simulink model "VCU_CONTROL"  (R2026a)
settings: Solver=VariableStepAuto
undefined symbols (not defined in the file): VCU_torque_fall_rate, VCU_torque_rise_rate
settings Model: Creator=renil  LastModifiedBy=renil

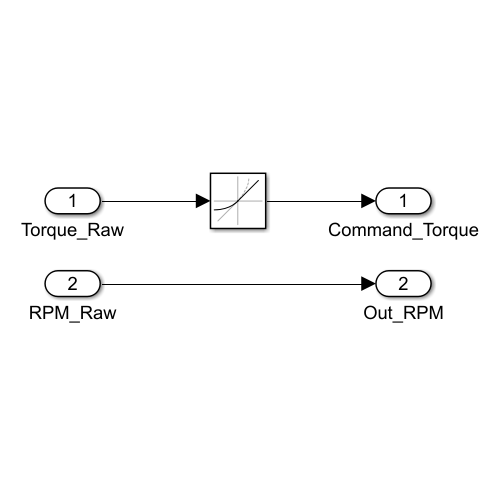
[thumbnail: Simulink's stored preview of the top-level diagram]
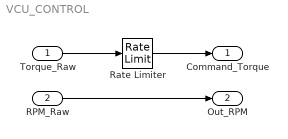
== system VCU_CONTROL ==
  Torque_Raw : Inport
  RPM_Raw : Inport  Port=2
  Rate Limiter : RateLimiter  RisingSlewLimit=VCU_torque_rise_rate  FallingSlewLimit=VCU_torque_fall_rate  SampleTimeMode=inherited
  Command_Torque : Outport
  Out_RPM : Outport  Port=2
  wires:
  RPM_Raw/1 -> Out_RPM/1
  Torque_Raw/1 -> Rate Limiter/1
  Rate Limiter/1 -> Command_Torque/1
